simulink model "DDCU_wxt_v02_forA_LabviewV03"  (R2014a)
settings: Solver=FixedStepDiscrete  StartTime=0.0  StopTime=50  FixedStep=0.0005  RelTol=1e-3
InitFcn:
  | Veh_Par_wxt
values from neighbouring files (symbols this model uses):
  ag_thr = 0.4*g    (= 3.924)    [Veh_Par_wxt.m]
  B = 2.25    [Veh_Par_wxt.m]
  bra_pre_em = 12    [Veh_Par_wxt.m]
  bra_pre_gz2 = 12/3    (= 4)    [Veh_Par_wxt.m]
  bra_pre_gz34 = 12/3    (= 4)    [Veh_Par_wxt.m]
  bra_pre_yd = 12/2    (= 6)    [Veh_Par_wxt.m]
  brakepre_dem_data = [0 1 2 3 4 5 6 7 8 9 10 11 12]    [Veh_Par_wxt.m]
  brakeTrq_dem_data = [0 218.198 436.396 654.594 872.792 1090.99 1309.188 1527.386 1745.584 1963.782 2181.98 2400.178 2618.376]    [Veh_Par_wxt.m]
  bratrq_max = 4*2618.376    (= 10473.504)    [Veh_Par_wxt.m]
  eff_tran = 0.75    [Veh_Par_wxt.m]
  G = Mass*g    (= 36297)    [Veh_Par_wxt.m]
  kd1 = 1    [Veh_Par_wxt.m]
  kd2 = 1    [Veh_Par_wxt.m]
  kd3 = 1    [Veh_Par_wxt.m]
  ki1 = 1    [Veh_Par_wxt.m]
  ki2 = 1    [Veh_Par_wxt.m]
  ki3 = 1    [Veh_Par_wxt.m]
  kp1 = 1    [Veh_Par_wxt.m]
  kp2 = 1    [Veh_Par_wxt.m]
  kp3 = 1    [Veh_Par_wxt.m]
  L = 3.12    [Veh_Par_wxt.m]
  premax = 12    [Veh_Par_wxt.m]
  Radius = 0.20    (= 0.2)    [Veh_Par_wxt.m]
  s_opt_yi_add = 0.05    [Veh_Par_wxt.m]
  s_opt_zhuan_add = 0.05    [Veh_Par_wxt.m]
  spd_map_mot = [0 100 200 300 360 400 500 600 700 800 900]*tras_ratio    [Veh_Par_wxt.m]
  spdmax = 900*tras_ratio    (= 5580)    [Veh_Par_wxt.m]
  speed_thr_park = 5/3.6/Radius*30/pi    (= 66.3145596216)    [Veh_Par_wxt.m]
  tras_ratio = 6.2    [Veh_Par_wxt.m]
  trq_map_mot = [1200 1200 1200 1200 1200 1080 864 720 617 540 480]/tras_ratio    [Veh_Par_wxt.m]
  trqmax = 80    [Veh_Par_wxt.m]
  trqmax_yd = 200    [Veh_Par_wxt.m]
  v_thr1_b = 5    [Veh_Par_wxt.m]
  v_thr2_b = 20    [Veh_Par_wxt.m]
  v_thr_park = 5    [Veh_Par_wxt.m]
undefined symbols (not defined in the file or in its folder): DiscIntNeverNeededParam
libraries: simulink x231, ec5744lib x19
(part 4 of 16)

== system DDCU_wxt_v02_forA_LabviewV03/OutputSignalProcess ==
  function : TriggerPort  TriggerType=function-call
  CANTransmit : ec5744lib/RapidECU_U3/04CANCommunication/CANTransmit  canmodule=0  canbuffer=8  canmessageid=hex2dec('0C01F001')  canmessagetype=Extended(29-bit ID)  datalength=8  sampletime=-1
  CANTransmit1 : ec5744lib/RapidECU_U3/04CANCommunication/CANTransmit  canmodule=0  canbuffer=9  canmessageid=hex2dec('0C01F002')  canmessagetype=Extended(29-bit ID)  datalength=8  sampletime=-1
  CANTransmit2 : ec5744lib/RapidECU_U3/04CANCommunication/CANTransmit  Commented=on  canmodule=0  canbuffer=10  canmessageid=hex2dec('804623A')  canmessagetype=Extended(29-bit ID)  datalength=8  sampletime=-1
  CANTransmit3 : ec5744lib/RapidECU_U3/04CANCommunication/CANTransmit  canmodule=0  canbuffer=11  canmessageid=hex2dec('0BF6EAF0')  canmessagetype=Extended(29-bit ID)  datalength=8  sampletime=-1
  Constant{,2..5} (5 alike) : Constant  SampleTime=-1
  Constant1 : Constant  Value=0  SampleTime=-1
  Data Store Read : DataStoreRead  DataStoreName=M1Enable
  Data Store Read1 : DataStoreRead  DataStoreName=M1Mode
  Data Store Read10 : DataStoreRead  DataStoreName=M3Drive
  Data Store Read11 : DataStoreRead  DataStoreName=M3TorqueSet
  Data Store Read12 : DataStoreRead  DataStoreName=M3SpeedSet
  Data Store Read13 : DataStoreRead  DialogController=Simulink.DDGSource  DataStoreName=M3TrqLimit
  Data Store Read14 : DataStoreRead  DataStoreName=M3SpeedLimit
  Data Store Read15 : DataStoreRead  DataStoreName=MCU2HeartBeat
  Data Store Read16 : DataStoreRead  DataStoreName=M2Enable
  Data Store Read17 : DataStoreRead  DataStoreName=M2Mode
  Data Store Read18 : DataStoreRead  DataStoreName=M2Drive
  Data Store Read19 : DataStoreRead  DataStoreName=M2TorqueSet
  Data Store Read2 : DataStoreRead  DataStoreName=M1Drive
  Data Store Read20 : DataStoreRead  DataStoreName=M2SpeedSet
  Data Store Read21 : DataStoreRead  DataStoreName=M2TrqLimit
  Data Store Read22 : DataStoreRead  DataStoreName=M2SpeedLimit
  Data Store Read23 : DataStoreRead  DataStoreName=M4Drive
  Data Store Read24 : DataStoreRead  DataStoreName=M4TorqueSet
  Data Store Read25 : DataStoreRead  DataStoreName=M4SpeedSet
  Data Store Read26 : DataStoreRead  DataStoreName=M4TrqLimit
  Data Store Read27 : DataStoreRead  DataStoreName=M4SpeedLimit
  Data Store Read28 : DataStoreRead  DataStoreName=M4Enable
  Data Store Read29 : DataStoreRead  DataStoreName=M4Mode
  Data Store Read3 : DataStoreRead  DataStoreName=M1TorqueSet
  Data Store Read30 : DataStoreRead  DataStoreName=bra_pre_l
  Data Store Read31 : DataStoreRead  DataStoreName=bra_pre_r
  Data Store Read32 : DataStoreRead  DataStoreName=M1InputVolt
  Data Store Read33 : DataStoreRead  DataStoreName=M4InputVolt
  Data Store Read34 : DataStoreRead  DataStoreName=M2InputVolt
  Data Store Read35 : DataStoreRead  DataStoreName=M3InputVolt
  Data Store Read4 : DataStoreRead  DataStoreName=M1SpeedSet
  Data Store Read5 : DataStoreRead  DataStoreName=M1TrqLimit
  Data Store Read6 : DataStoreRead  DataStoreName=M1SpeedLimit
  Data Store Read7 : DataStoreRead  DataStoreName=MCU1HeartBeat
  Data Store Read8 : DataStoreRead  DataStoreName=M3Enable
  Data Store Read9 : DataStoreRead  DataStoreName=M3Mode
  Data Type Conversion : DataTypeConversion
  Data Type Conversion1 : DataTypeConversion
  Ground : Ground  Commented=on
  Switch{,1..3} (4 alike) : Switch  Criteria=u2 > Threshold  Threshold=330
  Terminator{,1,3..11} (11 alike) : Terminator
  Terminator2 : Terminator  Commented=on
  VCU_ESC : Subsystem
  VCU_MCU1 : Subsystem
  VCU_MCU1_replace : Subsystem  Commented=on
  VCU_MCU2 : Subsystem
  VCU_MCU2_replace : Subsystem  Commented=on
  VCU_Park : Subsystem  Commented=on
  wires:
  Ground/1 -> VCU_Park/1(ParkEnable_in)
  Constant/1 -> Data Type Conversion/1
  VCU_MCU1/1(output) -> CANTransmit/1
  CANTransmit/1 -> Terminator/1
  VCU_MCU2/1(output) -> CANTransmit1/1
  CANTransmit1/1 -> Terminator1/1
  VCU_Park/1(output) -> CANTransmit2/1
  CANTransmit2/1 -> Terminator2/1
  VCU_ESC/1(output) -> CANTransmit3/1
  CANTransmit3/1 -> Terminator3/1
  Data Store Read4/1 -> Terminator4/1
  Data Store Read5/1 -> Terminator5/1
  Data Store Read20/1 -> Terminator6/1
  Data Store Read21/1 -> Terminator7/1
  Data Store Read12/1 -> Terminator8/1
  Data Store Read13/1 -> Terminator9/1
  Data Store Read25/1 -> Terminator10/1
  Data Store Read26/1 -> Terminator11/1
  Data Store Read14/1 -> VCU_MCU2/5(M3SpeedLimit_in)
  Data Store Read11/1 -> VCU_MCU2/4(M3TorqueSet_in)  "M3TorqueSet"
  Data Store Read15/1 -> VCU_MCU2/11(MCU2HeartBeat_in)
  Data Store Read27/1 -> VCU_MCU2/10(M4SpeedLimit_in)
  Data Store Read10/1 -> VCU_MCU2/3(M3Drive_in)  "M3Drive"
  Switch2/1 -> VCU_MCU2/1(M3Enable_in)  "M3Enable1"
  Data Store Read9/1 -> VCU_MCU2/2(M3Mode_in)  "M3Mode"
  Data Store Read24/1 -> VCU_MCU2/9(M4TorqueSet_in)  "M4TorqueSet"
  Data Store Read23/1 -> VCU_MCU2/8(M4Drive_in)  "M4Drive"
  Data Store Read29/1 -> VCU_MCU2/7(M4Mode_in)  "M4Mode"
  Data Store Read31/1 -> VCU_ESC/4(VVMS_BrkPSetRi_MPa_in)  "bra_pre_r"
  Data Store Read30/1 -> VCU_ESC/3(VVMS_BrkPSetLe_MPa_in)  "bra_pre_l"
  Constant1/1 -> Data Type Conversion1/1
  Data Type Conversion/1 -> VCU_ESC/1(VVMS_BrkSts_flg_in)
  Data Type Conversion1/1 -> VCU_ESC/2(VVMS_ParkSts_flg_in)
  Data Store Read7/1 -> VCU_MCU1/11(MCU1HeartBeat_in)
  Data Store Read19/1 -> VCU_MCU1/9(M2TorqueSet_in)  "M2TorqueSet"
  Data Store Read3/1 -> VCU_MCU1/4(M1TorqueSet_in)  "M1TorqueSet"
  Data Store Read6/1 -> VCU_MCU1/5(M1SpeedLimit_in)
  Data Store Read22/1 -> VCU_MCU1/10(M2SpeedLimit_in)
  Switch1/1 -> VCU_MCU1/6(M2Enable_in)  "M2Enable1"
  Data Store Read1/1 -> VCU_MCU1/2(M1Mode_in)  "M1Mode"
  Data Store Read18/1 -> VCU_MCU1/8(M2Drive_in)  "M2Drive"
  Data Store Read2/1 -> VCU_MCU1/3(M1Drive_in)  "M1Drive"
  Data Store Read17/1 -> VCU_MCU1/7(M2Mode_in)  "M2Mode"
  Data Store Read32/1 -> Switch/2
  Constant2/1 -> Switch/3
  Data Store Read/1 -> Switch/1
  Switch/1 -> VCU_MCU1/1(M1Enable_in)  "M1Enable1"
  Data Store Read34/1 -> Switch1/2
  Constant3/1 -> Switch1/3
  Data Store Read16/1 -> Switch1/1
  Data Store Read35/1 -> Switch2/2
  Constant4/1 -> Switch2/3
  Data Store Read8/1 -> Switch2/1
  Data Store Read33/1 -> Switch3/2
  Constant5/1 -> Switch3/3
  Data Store Read28/1 -> Switch3/1
  Switch3/1 -> VCU_MCU2/6(M4Enable_in)  "M4Enable1"

== system DDCU_wxt_v02_forA_LabviewV03/Data_Input/Function-Call Subsystem ==
  In1 : Inport
  In2 : Inport  Port=2
  function : TriggerPort  TriggerType=function-call
  ddcu1_ddcu2 : Subsystem
  brake_emerg : Outport
  steer_dem : Outport  Port=2
  mode_dem : Outport  Port=3
  brake_dem : Outport  Port=4
  acc_dem : Outport  Port=5
  wires:
  In1/1 -> ddcu1_ddcu2/Enable
  In2/1 -> ddcu1_ddcu2/1(input)
  ddcu1_ddcu2/3(mode_dem_Out) -> mode_dem/1
  ddcu1_ddcu2/2(steer_dem_Out) -> steer_dem/1
  ddcu1_ddcu2/4(brake_dem_Out) -> brake_dem/1
  ddcu1_ddcu2/1(brake_emerg_Out) -> brake_emerg/1
  ddcu1_ddcu2/5(acc_dem_Out) -> acc_dem/1

== system DDCU_wxt_v02_forA_LabviewV03/Data_Input/Function-Call Subsystem2 ==
  In1 : Inport
  In2 : Inport  Port=2
  function : TriggerPort  TriggerType=function-call
  ESC_VCU : Subsystem
  VESC_BrkPMa_MPa : Outport
  VESC_BrkPSetRi_MPa : Outport  Port=2
  VESC_BrkPSetLe_MPa : Outport  Port=3
  VESC_BrkFlt_enum : Outport  Port=4
  VESC_HotSts_flg : Outport  Port=5
  VESC_BrkReq_flg : Outport  Port=6
  VESC_ParkReq_flg : Outport  Port=7
  VESC_BrkPRi_MPa : Outport  Port=8
  VESC_BrkPLe_MPa : Outport  Port=9
  wires:
  ESC_VCU/1(VESC_BrkPMa_MPa_Out) -> VESC_BrkPMa_MPa/1
  ESC_VCU/2(VESC_BrkPSetRi_MPa_Out) -> VESC_BrkPSetRi_MPa/1
  ESC_VCU/3(VESC_BrkPSetLe_MPa_Out) -> VESC_BrkPSetLe_MPa/1
  ESC_VCU/4(VESC_BrkFlt_enum_Out) -> VESC_BrkFlt_enum/1
  ESC_VCU/5(VESC_HotSts_flg_Out) -> VESC_HotSts_flg/1
  ESC_VCU/6(VESC_BrkReq_flg_Out) -> VESC_BrkReq_flg/1
  ESC_VCU/7(VESC_ParkReq_flg_Out) -> VESC_ParkReq_flg/1
  ESC_VCU/8(VESC_BrkPRi_MPa_Out) -> VESC_BrkPRi_MPa/1
  ESC_VCU/9(VESC_BrkPLe_MPa_Out) -> VESC_BrkPLe_MPa/1
  In2/1 -> ESC_VCU/1(input)
  In1/1 -> ESC_VCU/Enable

== system DDCU_wxt_v02_forA_LabviewV03/Data_Input/HCU1_VCU ==
  In1 : Inport
  In2 : Inport  Port=2
  function : TriggerPort  TriggerType=function-call
  HCU1_VCU : Subsystem
  turn : Outport
  real_velocity : Outport  Port=2
  pwr_limit : Outport  Port=3
  break : Outport  Port=4
  acc : Outport  Port=5
  wires:
  In1/1 -> HCU1_VCU/Enable
  In2/1 -> HCU1_VCU/1(input)
  HCU1_VCU/3(pwr_limit_Out) -> pwr_limit/1
  HCU1_VCU/4(break_Out) -> break/1
  HCU1_VCU/2(real_velocity_Out) -> real_velocity/1
  HCU1_VCU/5(acc_Out) -> acc/1
  HCU1_VCU/1(turn_Out) -> turn/1

== system DDCU_wxt_v02_forA_LabviewV03/Data_Input/HCU1_VCU1 ==
  In1 : Inport
  In2 : Inport  Port=2
  function : TriggerPort  TriggerType=function-call
  MUC1_VCU1 : Subsystem
  spd_mot_rr : Outport
  spd_mot_rf : Outport  Port=2
  spd_mot_lr : Outport  Port=3
  spd_mot_lf : Outport  Port=4
  wires:
  In2/1 -> MUC1_VCU1/1(input)
  In1/1 -> MUC1_VCU1/Enable
  MUC1_VCU1/2(spd_mot_rf_Out) -> spd_mot_rf/1
  MUC1_VCU1/1(spd_mot_rr_Out) -> spd_mot_rr/1
  MUC1_VCU1/3(spd_mot_lr_Out) -> spd_mot_lr/1
  MUC1_VCU1/4(spd_mot_lf_Out) -> spd_mot_lf/1

== system DDCU_wxt_v02_forA_LabviewV03/Data_Input/HCU2_VCU ==
  In1 : Inport
  In2 : Inport  Port=2
  function : TriggerPort  TriggerType=function-call
  HCU2_VCU : Subsystem
  zhuche : Outport
  zhongxinzhuanxiang : Outport  Port=2
  qianjin : Outport  Port=3
  kongdang : Outport  Port=4
  daodang : Outport  Port=5
  wires:
  In2/1 -> HCU2_VCU/1(input)
  In1/1 -> HCU2_VCU/Enable
  HCU2_VCU/2(zhongxinzhuanxiang_Out) -> zhongxinzhuanxiang/1
  HCU2_VCU/3(qianjin_Out) -> qianjin/1
  HCU2_VCU/1(zhuche_Out) -> zhuche/1
  HCU2_VCU/4(kongdang_Out) -> kongdang/1
  HCU2_VCU/5(daodang_Out) -> daodang/1

== system DDCU_wxt_v02_forA_LabviewV03/Data_Input/MCU1_VCU1 ==
  In1 : Inport
  In2 : Inport  Port=2
  function : TriggerPort  TriggerType=function-call
  MCU1_VCU1 : Subsystem
  M1InputVolt : Outport
  M1Speed : Outport  Port=2
  M1Direction : Outport  Port=3
  M1State : Outport  Port=4
  M1HeartBeat : Outport  Port=5
  M1Current : Outport  Port=6
  M1Torque : Outport  Port=7
  wires:
  In1/1 -> MCU1_VCU1/Enable
  MCU1_VCU1/2(M1Speed_Out) -> M1Speed/1
  MCU1_VCU1/3(M1Direction_Out) -> M1Direction/1
  MCU1_VCU1/4(M1State_Out) -> M1State/1
  MCU1_VCU1/1(M1InputVolt_Out) -> M1InputVolt/1
  MCU1_VCU1/5(M1HeartBeat_Out) -> M1HeartBeat/1
  MCU1_VCU1/6(M1Current_Out) -> M1Current/1
  MCU1_VCU1/7(M1Torque_Out) -> M1Torque/1
  In2/1 -> MCU1_VCU1/1(input)

== system DDCU_wxt_v02_forA_LabviewV03/Data_Input/MCU1_VCU2 ==
  In1 : Inport
  In2 : Inport  Port=2
  function : TriggerPort  TriggerType=function-call
  MCU1_VCU2 : Subsystem
  M1FaultGrade : Outport
  M1FaultCode : Outport  Port=2
  M1TqLimit : Outport  Port=3
  M1IGBTTemp : Outport  Port=4
  M1Temp : Outport  Port=5
  wires:
  In1/1 -> MCU1_VCU2/Enable
  In2/1 -> MCU1_VCU2/1(input)
  MCU1_VCU2/2(M1FaultCode_Out) -> M1FaultCode/1
  MCU1_VCU2/3(M1TqLimit_Out) -> M1TqLimit/1
  MCU1_VCU2/1(M1FaultGrade_Out) -> M1FaultGrade/1
  MCU1_VCU2/4(M1IGBTTemp_Out) -> M1IGBTTemp/1
  MCU1_VCU2/5(M1Temp_Out) -> M1Temp/1

== system DDCU_wxt_v02_forA_LabviewV03/Data_Input/MCU1_VCU3 ==
  In1 : Inport
  In2 : Inport  Port=2
  function : TriggerPort  TriggerType=function-call
  MCU1_VCU3 : Subsystem
  M2InputVolt : Outport
  M2Speed : Outport  Port=2
  M2Direction : Outport  Port=3
  M2State : Outport  Port=4
  M2HeartBeat : Outport  Port=5
  M2Current : Outport  Port=6
  M2Torque : Outport  Port=7
  wires:
  In2/1 -> MCU1_VCU3/1(input)
  In1/1 -> MCU1_VCU3/Enable
  MCU1_VCU3/3(M2Direction_Out) -> M2Direction/1
  MCU1_VCU3/6(M2Current_Out) -> M2Current/1
  MCU1_VCU3/5(M2HeartBeat_Out) -> M2HeartBeat/1
  MCU1_VCU3/1(M2InputVolt_Out) -> M2InputVolt/1
  MCU1_VCU3/2(M2Speed_Out) -> M2Speed/1
  MCU1_VCU3/4(M2State_Out) -> M2State/1
  MCU1_VCU3/7(M2Torque_Out) -> M2Torque/1

== system DDCU_wxt_v02_forA_LabviewV03/Data_Input/MCU1_VCU4 ==
  In1 : Inport
  In2 : Inport  Port=2
  function : TriggerPort  TriggerType=function-call
  MCU1_VCU4 : Subsystem
  M2FaultGrade : Outport
  M2FaultCode : Outport  Port=2
  M2TqLimit : Outport  Port=3
  M2IGBTTemp : Outport  Port=4
  M2Temp : Outport  Port=5
  wires:
  In1/1 -> MCU1_VCU4/Enable
  In2/1 -> MCU1_VCU4/1(input)
  MCU1_VCU4/5(M2Temp_Out) -> M2Temp/1
  MCU1_VCU4/4(M2IGBTTemp_Out) -> M2IGBTTemp/1
  MCU1_VCU4/3(M2TqLimit_Out) -> M2TqLimit/1
  MCU1_VCU4/1(M2FaultGrade_Out) -> M2FaultGrade/1
  MCU1_VCU4/2(M2FaultCode_Out) -> M2FaultCode/1

== system DDCU_wxt_v02_forA_LabviewV03/Data_Input/MCU2_VCU1 ==
  In1 : Inport
  In2 : Inport  Port=2
  function : TriggerPort  TriggerType=function-call
  MCU2_VCU1 : Subsystem
  M3InputVolt : Outport
  M3Speed : Outport  Port=2
  M3Direction : Outport  Port=3
  M3State : Outport  Port=4
  M3HeartBeat : Outport  Port=5
  M3Current : Outport  Port=6
  M3Torque : Outport  Port=7
  wires:
  In1/1 -> MCU2_VCU1/Enable
  In2/1 -> MCU2_VCU1/1(input)
  MCU2_VCU1/7(M3Torque_Out) -> M3Torque/1
  MCU2_VCU1/6(M3Current_Out) -> M3Current/1
  MCU2_VCU1/5(M3HeartBeat_Out) -> M3HeartBeat/1
  MCU2_VCU1/4(M3State_Out) -> M3State/1
  MCU2_VCU1/3(M3Direction_Out) -> M3Direction/1
  MCU2_VCU1/2(M3Speed_Out) -> M3Speed/1
  MCU2_VCU1/1(M3InputVolt_Out) -> M3InputVolt/1

== system DDCU_wxt_v02_forA_LabviewV03/Data_Input/MCU2_VCU2 ==
  In1 : Inport
  In2 : Inport  Port=2
  function : TriggerPort  TriggerType=function-call
  MCU2_VCU2 : Subsystem
  M3FaultGrade : Outport
  M3FaultCode : Outport  Port=2
  M3TqLimit : Outport  Port=3
  M3IGBTTemp : Outport  Port=4
  M3Temp : Outport  Port=5
  wires:
  In1/1 -> MCU2_VCU2/Enable
  In2/1 -> MCU2_VCU2/1(input)
  MCU2_VCU2/2(M3FaultCode_Out) -> M3FaultCode/1
  MCU2_VCU2/1(M3FaultGrade_Out) -> M3FaultGrade/1
  MCU2_VCU2/3(M3TqLimit_Out) -> M3TqLimit/1
  MCU2_VCU2/4(M3IGBTTemp_Out) -> M3IGBTTemp/1
  MCU2_VCU2/5(M3Temp_Out) -> M3Temp/1

== system DDCU_wxt_v02_forA_LabviewV03/Data_Input/MCU2_VCU3 ==
  In1 : Inport
  In2 : Inport  Port=2
  function : TriggerPort  TriggerType=function-call
  MCU2_VCU3 : Subsystem
  M4InputVolt : Outport
  M4Speed : Outport  Port=2
  M4Direction : Outport  Port=3
  M4State : Outport  Port=4
  M4HeartBeat : Outport  Port=5
  M4Current : Outport  Port=6
  M4Torque : Outport  Port=7
  wires:
  In1/1 -> MCU2_VCU3/Enable
  In2/1 -> MCU2_VCU3/1(input)
  MCU2_VCU3/2(M4Speed_Out) -> M4Speed/1
  MCU2_VCU3/3(M4Direction_Out) -> M4Direction/1
  MCU2_VCU3/1(M4InputVolt_Out) -> M4InputVolt/1
  MCU2_VCU3/4(M4State_Out) -> M4State/1
  MCU2_VCU3/5(M4HeartBeat_Out) -> M4HeartBeat/1
  MCU2_VCU3/6(M4Current_Out) -> M4Current/1
  MCU2_VCU3/7(M4Torque_Out) -> M4Torque/1

== system DDCU_wxt_v02_forA_LabviewV03/Data_Input/MCU2_VCU4 ==
  In1 : Inport
  In2 : Inport  Port=2
  function : TriggerPort  TriggerType=function-call
  MCU2_VCU4 : Subsystem
  M4FaultGrade : Outport
  M4FaultCode : Outport  Port=2
  M4TqLimit : Outport  Port=3
  M4IGBTTemp : Outport  Port=4
  M4Temp : Outport  Port=5
  wires:
  In1/1 -> MCU2_VCU4/Enable
  In2/1 -> MCU2_VCU4/1(input)
  MCU2_VCU4/5(M4Temp_Out) -> M4Temp/1
  MCU2_VCU4/4(M4IGBTTemp_Out) -> M4IGBTTemp/1
  MCU2_VCU4/3(M4TqLimit_Out) -> M4TqLimit/1
  MCU2_VCU4/1(M4FaultGrade_Out) -> M4FaultGrade/1
  MCU2_VCU4/2(M4FaultCode_Out) -> M4FaultCode/1

== system DDCU_wxt_v02_forA_LabviewV03/InputSignalProcess/Battery ==
  pwr_dis_bat : Inport
  pwr_chg_bat : Inport  Port=2
  Bus Creator : BusCreator  Inputs=2
  Bat : Outport
  wires:
  pwr_dis_bat/1 -> Bus Creator/1  "pwr_dis_bat"
  Bus Creator/1 -> Bat/1  "Bat"
  pwr_chg_bat/1 -> Bus Creator/2  "pwr_chg_bat"

== system DDCU_wxt_v02_forA_LabviewV03/InputSignalProcess/BraSystem ==
  BraPre_act_l : Inport
  BraPre_act_r : Inport  Port=2
  Bus Creator : BusCreator  Inputs=2
  BraPre : Outport
  wires:
  BraPre_act_l/1 -> Bus Creator/1  "BraPre_act"
  Bus Creator/1 -> BraPre/1  "BraPre"
  BraPre_act_r/1 -> Bus Creator/2  "BraPre_act_r"

== system DDCU_wxt_v02_forA_LabviewV03/InputSignalProcess/DriveMotor ==
  speed_act_lf : Inport
  trq_act_lf : Inport  Port=2
  trqlimU_dig_lf : Inport  Port=3
  trqlimL_dig_lf : Inport  Port=4
  guzhang_lf : Inport  Port=5
  speed_act_lr : Inport  Port=6
  trq_act_lr : Inport  Port=7
  trqlimU_dig_lr : Inport  Port=8
  trqlimL_dig_lr : Inport  Port=9
  guzhang_lr : Inport  Port=10
  speed_act_rf : Inport  Port=11
  trq_act_rf : Inport  Port=12
  trqlimU_dig_rf : Inport  Port=13
  trqlimL_dig_rf : Inport  Port=14
  guzhang_rf : Inport  Port=15
  speed_act_rr : Inport  Port=16
  trq_act_rr : Inport  Port=17
  trqlimU_dig_rr : Inport  Port=18
  trqlimL_dig_rr : Inport  Port=19
  guzhang_rr : Inport  Port=20
  Bus Creator : BusCreator  Inputs=20
  DriveMotor : Outport
  wires:
  Bus Creator/1 -> DriveMotor/1  "DriveMotor"
  trqlimL_dig_lr/1 -> Bus Creator/9  "trqlimL_dig_lr"
  trq_act_lf/1 -> Bus Creator/2  "trq_act_lf"
  trq_act_lr/1 -> Bus Creator/7  "trq_act_lr"
  trqlimL_dig_lf/1 -> Bus Creator/4  "trqlimL_dig_lf"
  trqlimU_dig_lf/1 -> Bus Creator/3  "trqlimU_dig_lf"
  trqlimU_dig_lr/1 -> Bus Creator/8  "trqlimU_dig_lr"
  speed_act_lf/1 -> Bus Creator/1  "speed_act_lf"
  speed_act_lr/1 -> Bus Creator/6  "speed_act_lr"
  guzhang_rf/1 -> Bus Creator/15  "guzhang_rf"
  guzhang_lf/1 -> Bus Creator/5  "guzhang_lf"
  guzhang_lr/1 -> Bus Creator/10  "guzhang_lr"
  speed_act_rf/1 -> Bus Creator/11  "speed_act_rf"
  guzhang_rr/1 -> Bus Creator/20  "guzhang_rr"
  trq_act_rf/1 -> Bus Creator/12  "trq_act_rf"
  speed_act_rr/1 -> Bus Creator/16  "speed_act_rr"
  trqlimL_dig_rf/1 -> Bus Creator/14  "trqlimL_dig_rf"
  trq_act_rr/1 -> Bus Creator/17  "trq_act_rr"
  trqlimL_dig_rr/1 -> Bus Creator/19  "trqlimL_dig_rr"
  trqlimU_dig_rf/1 -> Bus Creator/13  "trqlimU_dig_rf"
  trqlimU_dig_rr/1 -> Bus Creator/18  "trqlimU_dig_rr"

== system DDCU_wxt_v02_forA_LabviewV03/InputSignalProcess/IMU ==
  v_act : Inport
  dis_east : Inport  Port=2
  dis_north : Inport  Port=3
  dis_sky : Inport  Port=4
  hangxiangangle : Inport  Port=5
  fuyangangle : Inport  Port=6
  henggunangle : Inport  Port=7
  acc_x : Inport  Port=8
  acc_y : Inport  Port=9
  acc_z : Inport  Port=10
  jiaosudu_x : Inport  Port=11
  jiaosudu_y : Inport  Port=12
  jiaosudu_z : Inport  Port=13
  Bus Creator : BusCreator  Inputs=13
  IMU : Outport
  wires:
  Bus Creator/1 -> IMU/1  "IMU"
  dis_east/1 -> Bus Creator/2  "dis_east"
  hangxiangangle/1 -> Bus Creator/5  "hangxiangangle"
  dis_north/1 -> Bus Creator/3  "dis_north"
  dis_sky/1 -> Bus Creator/4  "dis_sky"
  fuyangangle/1 -> Bus Creator/6  "fuyangangle"
  acc_y/1 -> Bus Creator/9  "acc_y"
  henggunangle/1 -> Bus Creator/7  "henggunangle"
  acc_x/1 -> Bus Creator/8  "acc_x"
  acc_z/1 -> Bus Creator/10  "acc_z"
  jiaosudu_z/1 -> Bus Creator/13  "jiaosudu_z"
  jiaosudu_x/1 -> Bus Creator/11  "jiaosudu_x"
  jiaosudu_y/1 -> Bus Creator/12  "jiaosudu_y"
  v_act/1 -> Bus Creator/1  "v_act"

== system DDCU_wxt_v02_forA_LabviewV03/InputSignalProcess/Subsystem ==
  zhuche : Inport
  zhongxinzhuanxiang : Inport  Port=2
  qianjin : Inport  Port=3
  kongdang : Inport  Port=4
  daodang : Inport  Port=5
  MATLAB Function : MATLAB Function  TreatAsAtomicUnit=on
  mode_dem : Outport
  wires:
  MATLAB Function/1(mode_dem) -> mode_dem/1
  zhuche/1 -> MATLAB Function/1(zhuche)
  zhongxinzhuanxiang/1 -> MATLAB Function/2(zhongxinzhuanxiang)
  qianjin/1 -> MATLAB Function/3(qianjin)
  kongdang/1 -> MATLAB Function/4(kongdang)
  daodang/1 -> MATLAB Function/5(daodang)

== system DDCU_wxt_v02_forA_LabviewV03/InputSignalProcess/Suspension ==
  location_center : Inport
  Bus Creator : BusCreator  Inputs=1
  Center_of_Mass : Outport
  wires:
  Bus Creator/1 -> Center_of_Mass/1  "Center_of_Mass"
  location_center/1 -> Bus Creator/1  "location_center"

== system DDCU_wxt_v02_forA_LabviewV03/InputSignalProcess/YaoKong ==
  note: 上坡辅助系统(Hill-start Assist Control，HAC)
  mode_dem : Inport
  acc_dem : Inport  Port=2
  steer_dem : Inport  Port=3
  brake_dem : Inport  Port=4
  brake_emerg : Inport  Port=5
  HAC : Inport  Port=6
  Bus Creator : BusCreator  Inputs=6
  YaoKong_dem : Outport
  wires:
  steer_dem/1 -> Bus Creator/3  "steer_dem"
  acc_dem/1 -> Bus Creator/2  "acc_dem"
  brake_dem/1 -> Bus Creator/4  "brake_dem"
  mode_dem/1 -> Bus Creator/1  "mode_dem"
  Bus Creator/1 -> YaoKong_dem/1  "YaoKong"
  brake_emerg/1 -> Bus Creator/5  "brake_emerg"
  HAC/1 -> Bus Creator/6  "HAC"

== system DDCU_wxt_v02_forA_LabviewV03/MainControl/SendOutPrepare ==
  com_dem : Inport
  Data Store Write : DataStoreWrite  DataStoreName=M1Enable
  Data Store Write1 : DataStoreWrite  DataStoreName=M1Mode
  Data Store Write10 : DataStoreWrite  DataStoreName=M3Drive
  Data Store Write11 : DataStoreWrite  DataStoreName=M3TorqueSet
  Data Store Write12 : DataStoreWrite  DataStoreName=M3SpeedSet
  Data Store Write13 : DataStoreWrite  DialogController=Simulink.DDGSource  DataStoreName=M3TrqLimit
  Data Store Write14 : DataStoreWrite  DataStoreName=M3SpeedLimit
  Data Store Write15 : DataStoreWrite  DataStoreName=MCU2HeartBeat
  Data Store Write16 : DataStoreWrite  DataStoreName=M2Enable
  Data Store Write17 : DataStoreWrite  DataStoreName=M2Mode
  Data Store Write18 : DataStoreWrite  DataStoreName=M2Drive
  Data Store Write19 : DataStoreWrite  DataStoreName=M2TorqueSet
  Data Store Write2 : DataStoreWrite  DataStoreName=M1Drive
  Data Store Write20 : DataStoreWrite  DataStoreName=M2SpeedSet
  Data Store Write21 : DataStoreWrite  DataStoreName=M2TrqLimit
  Data Store Write22 : DataStoreWrite  DataStoreName=M2SpeedLimit
  Data Store Write23 : DataStoreWrite  DataStoreName=M4Drive
  Data Store Write24 : DataStoreWrite  DataStoreName=M4TorqueSet
  Data Store Write25 : DataStoreWrite  DataStoreName=M4SpeedSet
  Data Store Write26 : DataStoreWrite  DataStoreName=M4TrqLimit
  Data Store Write27 : DataStoreWrite  DataStoreName=M4SpeedLimit
  Data Store Write28 : DataStoreWrite  DataStoreName=M4Enable
  Data Store Write29 : DataStoreWrite  DataStoreName=M4Mode
  Data Store Write3 : DataStoreWrite  DataStoreName=M1TorqueSet
  Data Store Write30 : DataStoreWrite  DataStoreName=bra_pre_l
  Data Store Write31 : DataStoreWrite  DataStoreName=bra_pre_r
  Data Store Write4 : DataStoreWrite  DataStoreName=M1SpeedSet
  Data Store Write5 : DataStoreWrite  DataStoreName=M1TrqLimit
  Data Store Write6 : DataStoreWrite  DataStoreName=M1SpeedLimit
  Data Store Write7 : DataStoreWrite  DataStoreName=MCU1HeartBeat
  Data Store Write8 : DataStoreWrite  DataStoreName=M3Enable
  Data Store Write9 : DataStoreWrite  DataStoreName=M3Mode
  Demux : Demux  Outputs=6
  Demux1 : Demux  Outputs=8
  Demux2 : Demux  Outputs=8
  Demux3 : Demux  Outputs=7
  Demux4 : Demux  Outputs=7
  Scope{,1..3} (4 alike) : Scope
      Scope2 settings: SaveName=ScopeData2
      Scope3 settings: SaveName=ScopeData3
  wires:
  Demux/1 -> Demux1/1
  Demux/2 -> Demux2/1
  Demux/3 -> Demux3/1
  Demux/4 -> Demux4/1
  Demux1/3 -> Data Store Write2/1
  Demux1/4 -> Scope/1, Data Store Write3/1
  Demux1/2 -> Data Store Write1/1
  Demux1/5 -> Data Store Write4/1
  Demux1/6 -> Data Store Write5/1
  Demux1/1 -> Data Store Write/1
  Demux1/7 -> Data Store Write6/1
  Demux1/8 -> Data Store Write7/1
  Demux2/7 -> Data Store Write14/1
  Demux2/6 -> Data Store Write13/1
  Demux2/1 -> Data Store Write8/1
  Demux2/8 -> Data Store Write15/1
  Demux2/5 -> Data Store Write12/1
  Demux2/2 -> Data Store Write9/1
  Demux2/4 -> Scope1/1, Data Store Write11/1
  Demux2/3 -> Data Store Write10/1
  Demux3/1 -> Data Store Write16/1
  Demux3/6 -> Data Store Write21/1
  Demux3/7 -> Data Store Write22/1
  Demux3/5 -> Data Store Write20/1
  Demux3/4 -> Scope2/1, Data Store Write19/1
  Demux3/2 -> Data Store Write17/1
  Demux3/3 -> Data Store Write18/1
  Demux4/1 -> Data Store Write28/1
  Demux4/2 -> Data Store Write29/1
  Demux4/3 -> Data Store Write23/1
  Demux4/4 -> Scope3/1, Data Store Write24/1
  Demux4/5 -> Data Store Write25/1
  Demux4/6 -> Data Store Write26/1
  Demux4/7 -> Data Store Write27/1
  Demux/5 -> Data Store Write30/1
  Demux/6 -> Data Store Write31/1
  com_dem/1 -> Demux/1

== system DDCU_wxt_v02_forA_LabviewV03/MainControl/mode_control ==
  mode_dem_out : Inport
  Signals : Inport  Port=2
  Multiport Switch : MultiPortSwitch  DataPortOrder=Zero-based contiguous  Inputs=6
  Park : Subsystem  TreatAsAtomicUnit=on
  Switch Case : SwitchCase  CaseConditions={0,1,2,3,4,5}  ShowDefaultCase=off
  backward : Subsystem  TreatAsAtomicUnit=on
  center_steer : Subsystem  TreatAsAtomicUnit=on
  emergency_stop : Subsystem  TreatAsAtomicUnit=on
  forward : Subsystem  TreatAsAtomicUnit=on
  neutral : Subsystem  TreatAsAtomicUnit=on
  com_dem : Outport
  wires:
  mode_dem_out/1 -> Multiport Switch/1, Switch Case/1  "mode_dem_out"
  Signals/1 -> backward/1(Signals), emergency_stop/1(Signals), center_steer/1(Signals), neutral/1(Signals), forward/1(Signals), Park/1(Signals)
  Switch Case/1 -> Park/Action
  Switch Case/6 -> emergency_stop/Action
  Switch Case/5 -> center_steer/Action
  Switch Case/4 -> backward/Action
  Switch Case/3 -> neutral/Action
  Switch Case/2 -> forward/Action
  Park/1(park_dem) -> Multiport Switch/2
  forward/1(forward_dem) -> Multiport Switch/3
  backward/1(backward_dem) -> Multiport Switch/5
  neutral/1(neutral_dem) -> Multiport Switch/4
  center_steer/1(center_steer_dem) -> Multiport Switch/6
  emergency_stop/1(emergency_stop_dem) -> Multiport Switch/7
  Multiport Switch/1 -> com_dem/1

== system DDCU_wxt_v02_forA_LabviewV03/MainControl/mode_switch ==
  note: 驻车转速
  note: 驻车车速阈值5km/h
  Signals : Inport
  Abs{,1..3} (4 alike) : Abs
  Bus Selector : BusSelector  OutputSignals=YaoKong.mode_dem,YaoKong.brake_emerg,DriveMotor.speed_act_lf,DriveMotor.speed_act_lr,DriveMotor.speed_act_rf,DriveMotor.speed_act_rr,IMU.v_act
  Constant1 : Constant  Value=v_thr_park  SampleTime=-1
  Constant2 : Constant  Value=speed_thr_park  SampleTime=-1
  Data Type Conversion : DataTypeConversion
  Data Type Conversion1 : DataTypeConversion
  Data Type Conversion2 : DataTypeConversion
  Memory : Memory  InheritSampleTime=on
  mode_switch : MATLAB Function  TreatAsAtomicUnit=on
  mode_dem_out : Outport
  wires:
  Memory/1 -> mode_switch/10(mode_dem_out_pre)
  Signals/1 -> Data Type Conversion/1
  Bus Selector/3 -> Abs/1  "<speed_act_lf>"
  Bus Selector/2 -> mode_switch/2(brake_emerg)  "<brake_emerg>"
  Bus Selector/1 -> mode_switch/1(mode_dem)  "<mode_dem>"
  Bus Selector/5 -> Abs2/1  "<speed_act_rf>"
  Bus Selector/4 -> Abs1/1  "<speed_act_lr>"
  Bus Selector/6 -> Abs3/1  "<speed_act_rr>"
  Bus Selector/7 -> mode_switch/7(v_act)  "<v_act>"
  mode_switch/1(mode_dem_out) -> mode_dem_out/1, Memory/1
  Constant2/1 -> Data Type Conversion2/1
  Constant1/1 -> Data Type Conversion1/1
  Abs/1 -> mode_switch/3(speed_act_lf)
  Abs1/1 -> mode_switch/4(speed_act_lr)
  Abs2/1 -> mode_switch/5(speed_act_rf)
  Abs3/1 -> mode_switch/6(speed_act_rr)
  Data Type Conversion/1 -> Bus Selector/1
  Data Type Conversion1/1 -> mode_switch/8(v_thr_park)
  Data Type Conversion2/1 -> mode_switch/9(speed_thr_park)

== system DDCU_wxt_v02_forA_LabviewV03/OutputSignalProcess/VCU_ESC ==
  VVMS_BrkSts_flg_in : Inport
  VVMS_ParkSts_flg_in : Inport  Port=2
  VVMS_BrkPSetLe_MPa_in : Inport  Port=3
  VVMS_BrkPSetRi_MPa_in : Inport  Port=4
  Conv{1..8} (8 alike) : DataTypeConversion
  VCU_ESC_DLC : Constant  Value=8  OutDataTypeStr=uint8
  VCU_ESC_DLC_Out : Terminator
  VCU_ESC_ID : Constant  Value=2364992240  OutDataTypeStr=single
  VCU_ESC_ID_Out : Terminator
  VCU_ESC_mux : Mux  Inputs=8
  VVMS_BrkPSetLe_MPa : Subsystem
  VVMS_BrkPSetRi_MPa : Subsystem
  VVMS_BrkSts_flg : Subsystem
  VVMS_ParkSts_flg : Subsystem
  or{1..8} (8 alike) : simulink/Logic and Bit Operations/Bitwise Operator  logicop=OR  UseBitMask=off  NumInputPorts=4  BitMask=bin2dec('11011001')  BitMaskRealWorld=Stored Integer
  output : Outport
  wires:
  VCU_ESC_mux/1 -> output/1
  VVMS_BrkSts_flg/1(output1) -> or1/1
  VVMS_BrkSts_flg/2(output2) -> or2/1
  VVMS_BrkSts_flg/3(output3) -> or3/1
  VVMS_BrkSts_flg/4(output4) -> or4/1
  VVMS_BrkSts_flg/5(output5) -> or5/1
  VVMS_BrkSts_flg/6(output6) -> or6/1
  VVMS_BrkSts_flg/7(output7) -> or7/1
  VVMS_BrkSts_flg/8(output8) -> or8/1
  VVMS_ParkSts_flg/1(output1) -> or1/2
  VVMS_ParkSts_flg/2(output2) -> or2/2
  VVMS_ParkSts_flg/3(output3) -> or3/2
  VVMS_ParkSts_flg/4(output4) -> or4/2
  VVMS_ParkSts_flg/5(output5) -> or5/2
  VVMS_ParkSts_flg/6(output6) -> or6/2
  VVMS_ParkSts_flg/7(output7) -> or7/2
  VVMS_ParkSts_flg/8(output8) -> or8/2
  VVMS_BrkPSetRi_MPa/1(output1) -> or1/3
  VVMS_BrkPSetRi_MPa/2(output2) -> or2/3
  VVMS_BrkPSetRi_MPa/3(output3) -> or3/3
  VVMS_BrkPSetRi_MPa/4(output4) -> or4/3
  VVMS_BrkPSetRi_MPa/5(output5) -> or5/3
  VVMS_BrkPSetRi_MPa/6(output6) -> or6/3
  VVMS_BrkPSetRi_MPa/7(output7) -> or7/3
  VVMS_BrkPSetRi_MPa/8(output8) -> or8/3
  VVMS_BrkPSetLe_MPa/1(output1) -> or1/4
  VVMS_BrkPSetLe_MPa/2(output2) -> or2/4
  VVMS_BrkPSetLe_MPa/3(output3) -> or3/4
  VVMS_BrkPSetLe_MPa/4(output4) -> or4/4
  VVMS_BrkPSetLe_MPa/5(output5) -> or5/4
  VVMS_BrkPSetLe_MPa/6(output6) -> or6/4
  VVMS_BrkPSetLe_MPa/7(output7) -> or7/4
  VVMS_BrkPSetLe_MPa/8(output8) -> or8/4
  or1/1 -> Conv1/1
  Conv1/1 -> VCU_ESC_mux/1
  or2/1 -> Conv2/1
  Conv2/1 -> VCU_ESC_mux/2
  or3/1 -> Conv3/1
  Conv3/1 -> VCU_ESC_mux/3
  or4/1 -> Conv4/1
  Conv4/1 -> VCU_ESC_mux/4
  or5/1 -> Conv5/1
  Conv5/1 -> VCU_ESC_mux/5
  or6/1 -> Conv6/1
  Conv6/1 -> VCU_ESC_mux/6
  or7/1 -> Conv7/1
  Conv7/1 -> VCU_ESC_mux/7
  or8/1 -> Conv8/1
  Conv8/1 -> VCU_ESC_mux/8
  VCU_ESC_ID/1 -> VCU_ESC_ID_Out/1
  VCU_ESC_DLC/1 -> VCU_ESC_DLC_Out/1
  VVMS_BrkSts_flg_in/1 -> VVMS_BrkSts_flg/1(VVMS_BrkSts_flg)
  VVMS_ParkSts_flg_in/1 -> VVMS_ParkSts_flg/1(VVMS_ParkSts_flg)
  VVMS_BrkPSetRi_MPa_in/1 -> VVMS_BrkPSetRi_MPa/1(VVMS_BrkPSetRi_MPa)
  VVMS_BrkPSetLe_MPa_in/1 -> VVMS_BrkPSetLe_MPa/1(VVMS_BrkPSetLe_MPa)

== system DDCU_wxt_v02_forA_LabviewV03/OutputSignalProcess/VCU_MCU1 ==
  M1Enable_in : Inport
  M1Mode_in : Inport  Port=2
  M1Drive_in : Inport  Port=3
  M1TorqueSet_in : Inport  Port=4
  M1SpeedLimit_in : Inport  Port=5
  M2Enable_in : Inport  Port=6
  M2Mode_in : Inport  Port=7
  M2Drive_in : Inport  Port=8
  M2TorqueSet_in : Inport  Port=9
  M2SpeedLimit_in : Inport  Port=10
  MCU1HeartBeat_in : Inport  Port=11
  Conv{1..8} (8 alike) : DataTypeConversion
  M1Drive : Subsystem
  M1Enable : Subsystem
  M1Mode : Subsystem
  M1SpeedLimit : Subsystem
  M1TorqueSet : Subsystem
  M2Drive : Subsystem
  M2Enable : Subsystem
  M2Mode : Subsystem
  M2SpeedLimit : Subsystem
  M2TorqueSet : Subsystem
  MCU1HeartBeat : Subsystem
  VCU_MCU1_DLC : Constant  Value=8  OutDataTypeStr=uint8
  VCU_MCU1_DLC_Out : Terminator
  VCU_MCU1_ID : Constant  Value=2348937217  OutDataTypeStr=single
  VCU_MCU1_ID_Out : Terminator
  VCU_MCU1_mux : Mux  Inputs=8
  or{1..8} (8 alike) : simulink/Logic and Bit Operations/Bitwise Operator  logicop=OR  UseBitMask=off  NumInputPorts=11  BitMask=bin2dec('11011001')  BitMaskRealWorld=Stored Integer
  output : Outport
  wires:
  VCU_MCU1_mux/1 -> output/1
  MCU1HeartBeat/1(output1) -> or1/1
  MCU1HeartBeat/2(output2) -> or2/1
  MCU1HeartBeat/3(output3) -> or3/1
  MCU1HeartBeat/4(output4) -> or4/1
  MCU1HeartBeat/5(output5) -> or5/1
  MCU1HeartBeat/6(output6) -> or6/1
  MCU1HeartBeat/7(output7) -> or7/1
  MCU1HeartBeat/8(output8) -> or8/1
  M2TorqueSet/1(output1) -> or1/2
  M2TorqueSet/2(output2) -> or2/2
  M2TorqueSet/3(output3) -> or3/2
  M2TorqueSet/4(output4) -> or4/2
  M2TorqueSet/5(output5) -> or5/2
  M2TorqueSet/6(output6) -> or6/2
  M2TorqueSet/7(output7) -> or7/2
  M2TorqueSet/8(output8) -> or8/2
  M2SpeedLimit/1(output1) -> or1/3
  M2SpeedLimit/2(output2) -> or2/3
  M2SpeedLimit/3(output3) -> or3/3
  M2SpeedLimit/4(output4) -> or4/3
  M2SpeedLimit/5(output5) -> or5/3
  M2SpeedLimit/6(output6) -> or6/3
  M2SpeedLimit/7(output7) -> or7/3
  M2SpeedLimit/8(output8) -> or8/3
  M2Mode/1(output1) -> or1/4
  M2Mode/2(output2) -> or2/4
  M2Mode/3(output3) -> or3/4
  M2Mode/4(output4) -> or4/4
  M2Mode/5(output5) -> or5/4
  M2Mode/6(output6) -> or6/4
  M2Mode/7(output7) -> or7/4
  M2Mode/8(output8) -> or8/4
  M2Enable/1(output1) -> or1/5
  M2Enable/2(output2) -> or2/5
  M2Enable/3(output3) -> or3/5
  M2Enable/4(output4) -> or4/5
  M2Enable/5(output5) -> or5/5
  M2Enable/6(output6) -> or6/5
  M2Enable/7(output7) -> or7/5
  M2Enable/8(output8) -> or8/5
  M2Drive/1(output1) -> or1/6
  M2Drive/2(output2) -> or2/6
  M2Drive/3(output3) -> or3/6
  M2Drive/4(output4) -> or4/6
  M2Drive/5(output5) -> or5/6
  M2Drive/6(output6) -> or6/6
  M2Drive/7(output7) -> or7/6
  M2Drive/8(output8) -> or8/6
  M1TorqueSet/1(output1) -> or1/7
  M1TorqueSet/2(output2) -> or2/7
  M1TorqueSet/3(output3) -> or3/7
  M1TorqueSet/4(output4) -> or4/7
  M1TorqueSet/5(output5) -> or5/7
  M1TorqueSet/6(output6) -> or6/7
  M1TorqueSet/7(output7) -> or7/7
  M1TorqueSet/8(output8) -> or8/7
  M1SpeedLimit/1(output1) -> or1/8
  M1SpeedLimit/2(output2) -> or2/8
  M1SpeedLimit/3(output3) -> or3/8
  M1SpeedLimit/4(output4) -> or4/8
  M1SpeedLimit/5(output5) -> or5/8
  M1SpeedLimit/6(output6) -> or6/8
  M1SpeedLimit/7(output7) -> or7/8
  M1SpeedLimit/8(output8) -> or8/8
  M1Mode/1(output1) -> or1/9
  M1Mode/2(output2) -> or2/9
  M1Mode/3(output3) -> or3/9
  M1Mode/4(output4) -> or4/9
  M1Mode/5(output5) -> or5/9
  M1Mode/6(output6) -> or6/9
  M1Mode/7(output7) -> or7/9
  M1Mode/8(output8) -> or8/9
  M1Enable/1(output1) -> or1/10
  M1Enable/2(output2) -> or2/10
  M1Enable/3(output3) -> or3/10
  M1Enable/4(output4) -> or4/10
  M1Enable/5(output5) -> or5/10
  M1Enable/6(output6) -> or6/10
  M1Enable/7(output7) -> or7/10
  M1Enable/8(output8) -> or8/10
  M1Drive/1(output1) -> or1/11
  M1Drive/2(output2) -> or2/11
  M1Drive/3(output3) -> or3/11
  M1Drive/4(output4) -> or4/11
  M1Drive/5(output5) -> or5/11
  M1Drive/6(output6) -> or6/11
  M1Drive/7(output7) -> or7/11
  M1Drive/8(output8) -> or8/11
  or1/1 -> Conv1/1
  Conv1/1 -> VCU_MCU1_mux/1
  or2/1 -> Conv2/1
  Conv2/1 -> VCU_MCU1_mux/2
  or3/1 -> Conv3/1
  Conv3/1 -> VCU_MCU1_mux/3
  or4/1 -> Conv4/1
  Conv4/1 -> VCU_MCU1_mux/4
  or5/1 -> Conv5/1
  Conv5/1 -> VCU_MCU1_mux/5
  or6/1 -> Conv6/1
  Conv6/1 -> VCU_MCU1_mux/6
  or7/1 -> Conv7/1
  Conv7/1 -> VCU_MCU1_mux/7
  or8/1 -> Conv8/1
  Conv8/1 -> VCU_MCU1_mux/8
  VCU_MCU1_ID/1 -> VCU_MCU1_ID_Out/1
  VCU_MCU1_DLC/1 -> VCU_MCU1_DLC_Out/1
  MCU1HeartBeat_in/1 -> MCU1HeartBeat/1(MCU1HeartBeat)
  M2TorqueSet_in/1 -> M2TorqueSet/1(M2TorqueSet)
  M2SpeedLimit_in/1 -> M2SpeedLimit/1(M2SpeedLimit)
  M2Mode_in/1 -> M2Mode/1(M2Mode)
  M2Enable_in/1 -> M2Enable/1(M2Enable)
  M2Drive_in/1 -> M2Drive/1(M2Drive)
  M1TorqueSet_in/1 -> M1TorqueSet/1(M1TorqueSet)
  M1SpeedLimit_in/1 -> M1SpeedLimit/1(M1SpeedLimit)
  M1Mode_in/1 -> M1Mode/1(M1Mode)
  M1Enable_in/1 -> M1Enable/1(M1Enable)
  M1Drive_in/1 -> M1Drive/1(M1Drive)

== system DDCU_wxt_v02_forA_LabviewV03/OutputSignalProcess/VCU_MCU1_replace ==
  M2SpeedSet_in : Inport
  M1SpeedSet_in : Inport  Port=2
  MCU1HeartBeat_in : Inport  Port=3
  M2SpeedLimit_in : Inport  Port=4
  M2Mode_in : Inport  Port=5
  M2Enable_in : Inport  Port=6
  M2Drive_in : Inport  Port=7
  M1SpeedLimit_in : Inport  Port=8
  M1Mode_in : Inport  Port=9
  M1Enable_in : Inport  Port=10
  M1Drive_in : Inport  Port=11
  Conv{1..8} (8 alike) : DataTypeConversion
  M1Drive : Subsystem
  M1Enable : Subsystem
  M1Mode : Subsystem
  M1SpeedLimit : Subsystem
  M1SpeedSet : Subsystem
  M2Drive : Subsystem
  M2Enable : Subsystem
  M2Mode : Subsystem
  M2SpeedLimit : Subsystem
  M2SpeedSet : Subsystem
  MCU1HeartBeat : Subsystem
  VCU_MCU1_replace_DLC : Constant  Value=8  OutDataTypeStr=uint8
  VCU_MCU1_replace_DLC_Out : Terminator
  VCU_MCU1_replace_ID : Constant  Value=2348937233  OutDataTypeStr=single
  VCU_MCU1_replace_ID_Out : Terminator
  VCU_MCU1_replace_mux : Mux  Inputs=8
  or{1..8} (8 alike) : simulink/Logic and Bit Operations/Bitwise Operator  logicop=OR  UseBitMask=off  NumInputPorts=11  BitMask=bin2dec('11011001')  BitMaskRealWorld=Stored Integer
  output : Outport
  wires:
  VCU_MCU1_replace_mux/1 -> output/1
  M2SpeedSet/1(output1) -> or1/1
  M2SpeedSet/2(output2) -> or2/1
  M2SpeedSet/3(output3) -> or3/1
  M2SpeedSet/4(output4) -> or4/1
  M2SpeedSet/5(output5) -> or5/1
  M2SpeedSet/6(output6) -> or6/1
  M2SpeedSet/7(output7) -> or7/1
  M2SpeedSet/8(output8) -> or8/1
  M1SpeedSet/1(output1) -> or1/2
  M1SpeedSet/2(output2) -> or2/2
  M1SpeedSet/3(output3) -> or3/2
  M1SpeedSet/4(output4) -> or4/2
  M1SpeedSet/5(output5) -> or5/2
  M1SpeedSet/6(output6) -> or6/2
  M1SpeedSet/7(output7) -> or7/2
  M1SpeedSet/8(output8) -> or8/2
  MCU1HeartBeat/1(output1) -> or1/3
  MCU1HeartBeat/2(output2) -> or2/3
  MCU1HeartBeat/3(output3) -> or3/3
  MCU1HeartBeat/4(output4) -> or4/3
  MCU1HeartBeat/5(output5) -> or5/3
  MCU1HeartBeat/6(output6) -> or6/3
  MCU1HeartBeat/7(output7) -> or7/3
  MCU1HeartBeat/8(output8) -> or8/3
  M2SpeedLimit/1(output1) -> or1/4
  M2SpeedLimit/2(output2) -> or2/4
  M2SpeedLimit/3(output3) -> or3/4
  M2SpeedLimit/4(output4) -> or4/4
  M2SpeedLimit/5(output5) -> or5/4
  M2SpeedLimit/6(output6) -> or6/4
  M2SpeedLimit/7(output7) -> or7/4
  M2SpeedLimit/8(output8) -> or8/4
  M2Mode/1(output1) -> or1/5
  M2Mode/2(output2) -> or2/5
  M2Mode/3(output3) -> or3/5
  M2Mode/4(output4) -> or4/5
  M2Mode/5(output5) -> or5/5
  M2Mode/6(output6) -> or6/5
  M2Mode/7(output7) -> or7/5
  M2Mode/8(output8) -> or8/5
  M2Enable/1(output1) -> or1/6
  M2Enable/2(output2) -> or2/6
  M2Enable/3(output3) -> or3/6
  M2Enable/4(output4) -> or4/6
  M2Enable/5(output5) -> or5/6
  M2Enable/6(output6) -> or6/6
  M2Enable/7(output7) -> or7/6
  M2Enable/8(output8) -> or8/6
  M2Drive/1(output1) -> or1/7
  M2Drive/2(output2) -> or2/7
  M2Drive/3(output3) -> or3/7
  M2Drive/4(output4) -> or4/7
  M2Drive/5(output5) -> or5/7
  M2Drive/6(output6) -> or6/7
  M2Drive/7(output7) -> or7/7
  M2Drive/8(output8) -> or8/7
  M1SpeedLimit/1(output1) -> or1/8
  M1SpeedLimit/2(output2) -> or2/8
  M1SpeedLimit/3(output3) -> or3/8
  M1SpeedLimit/4(output4) -> or4/8
  M1SpeedLimit/5(output5) -> or5/8
  M1SpeedLimit/6(output6) -> or6/8
  M1SpeedLimit/7(output7) -> or7/8
  M1SpeedLimit/8(output8) -> or8/8
  M1Mode/1(output1) -> or1/9
  M1Mode/2(output2) -> or2/9
  M1Mode/3(output3) -> or3/9
  M1Mode/4(output4) -> or4/9
  M1Mode/5(output5) -> or5/9
  M1Mode/6(output6) -> or6/9
  M1Mode/7(output7) -> or7/9
  M1Mode/8(output8) -> or8/9
  M1Enable/1(output1) -> or1/10
  M1Enable/2(output2) -> or2/10
  M1Enable/3(output3) -> or3/10
  M1Enable/4(output4) -> or4/10
  M1Enable/5(output5) -> or5/10
  M1Enable/6(output6) -> or6/10
  M1Enable/7(output7) -> or7/10
  M1Enable/8(output8) -> or8/10
  M1Drive/1(output1) -> or1/11
  M1Drive/2(output2) -> or2/11
  M1Drive/3(output3) -> or3/11
  M1Drive/4(output4) -> or4/11
  M1Drive/5(output5) -> or5/11
  M1Drive/6(output6) -> or6/11
  M1Drive/7(output7) -> or7/11
  M1Drive/8(output8) -> or8/11
  or1/1 -> Conv1/1
  Conv1/1 -> VCU_MCU1_replace_mux/1
  or2/1 -> Conv2/1
  Conv2/1 -> VCU_MCU1_replace_mux/2
  or3/1 -> Conv3/1
  Conv3/1 -> VCU_MCU1_replace_mux/3
  or4/1 -> Conv4/1
  Conv4/1 -> VCU_MCU1_replace_mux/4
  or5/1 -> Conv5/1
  Conv5/1 -> VCU_MCU1_replace_mux/5
  or6/1 -> Conv6/1
  Conv6/1 -> VCU_MCU1_replace_mux/6
  or7/1 -> Conv7/1
  Conv7/1 -> VCU_MCU1_replace_mux/7
  or8/1 -> Conv8/1
  Conv8/1 -> VCU_MCU1_replace_mux/8
  VCU_MCU1_replace_ID/1 -> VCU_MCU1_replace_ID_Out/1
  VCU_MCU1_replace_DLC/1 -> VCU_MCU1_replace_DLC_Out/1
  M2SpeedSet_in/1 -> M2SpeedSet/1(M2SpeedSet)
  M1SpeedSet_in/1 -> M1SpeedSet/1(M1SpeedSet)
  MCU1HeartBeat_in/1 -> MCU1HeartBeat/1(MCU1HeartBeat)
  M2SpeedLimit_in/1 -> M2SpeedLimit/1(M2SpeedLimit)
  M2Mode_in/1 -> M2Mode/1(M2Mode)
  M2Enable_in/1 -> M2Enable/1(M2Enable)
  M2Drive_in/1 -> M2Drive/1(M2Drive)
  M1SpeedLimit_in/1 -> M1SpeedLimit/1(M1SpeedLimit)
  M1Mode_in/1 -> M1Mode/1(M1Mode)
  M1Enable_in/1 -> M1Enable/1(M1Enable)
  M1Drive_in/1 -> M1Drive/1(M1Drive)

== system DDCU_wxt_v02_forA_LabviewV03/OutputSignalProcess/VCU_MCU2 ==
  M3Enable_in : Inport
  M3Mode_in : Inport  Port=2
  M3Drive_in : Inport  Port=3
  M3TorqueSet_in : Inport  Port=4
  M3SpeedLimit_in : Inport  Port=5
  M4Enable_in : Inport  Port=6
  M4Mode_in : Inport  Port=7
  M4Drive_in : Inport  Port=8
  M4TorqueSet_in : Inport  Port=9
  M4SpeedLimit_in : Inport  Port=10
  MCU2HeartBeat_in : Inport  Port=11
  Conv{1..8} (8 alike) : DataTypeConversion
  M3Drive : Subsystem
  M3Enable : Subsystem
  M3Mode : Subsystem
  M3SpeedLimit : Subsystem
  M3TorqueSet : Subsystem
  M4Drive : Subsystem
  M4Enable : Subsystem
  M4Mode : Subsystem
  M4SpeedLimit : Subsystem
  M4TorqueSet : Subsystem
  MCU2HeartBeat : Subsystem
  VCU_MCU2_DLC : Constant  Value=8  OutDataTypeStr=uint8
  VCU_MCU2_DLC_Out : Terminator
  VCU_MCU2_ID : Constant  Value=2348937218  OutDataTypeStr=single
  VCU_MCU2_ID_Out : Terminator
  VCU_MCU2_mux : Mux  Inputs=8
  or{1..8} (8 alike) : simulink/Logic and Bit Operations/Bitwise Operator  logicop=OR  UseBitMask=off  NumInputPorts=11  BitMask=bin2dec('11011001')  BitMaskRealWorld=Stored Integer
  output : Outport
  wires:
  VCU_MCU2_mux/1 -> output/1
  MCU2HeartBeat/1(output1) -> or1/1
  MCU2HeartBeat/2(output2) -> or2/1
  MCU2HeartBeat/3(output3) -> or3/1
  MCU2HeartBeat/4(output4) -> or4/1
  MCU2HeartBeat/5(output5) -> or5/1
  MCU2HeartBeat/6(output6) -> or6/1
  MCU2HeartBeat/7(output7) -> or7/1
  MCU2HeartBeat/8(output8) -> or8/1
  M4TorqueSet/1(output1) -> or1/2
  M4TorqueSet/2(output2) -> or2/2
  M4TorqueSet/3(output3) -> or3/2
  M4TorqueSet/4(output4) -> or4/2
  M4TorqueSet/5(output5) -> or5/2
  M4TorqueSet/6(output6) -> or6/2
  M4TorqueSet/7(output7) -> or7/2
  M4TorqueSet/8(output8) -> or8/2
  M4SpeedLimit/1(output1) -> or1/3
  M4SpeedLimit/2(output2) -> or2/3
  M4SpeedLimit/3(output3) -> or3/3
  M4SpeedLimit/4(output4) -> or4/3
  M4SpeedLimit/5(output5) -> or5/3
  M4SpeedLimit/6(output6) -> or6/3
  M4SpeedLimit/7(output7) -> or7/3
  M4SpeedLimit/8(output8) -> or8/3
  M4Mode/1(output1) -> or1/4
  M4Mode/2(output2) -> or2/4
  M4Mode/3(output3) -> or3/4
  M4Mode/4(output4) -> or4/4
  M4Mode/5(output5) -> or5/4
  M4Mode/6(output6) -> or6/4
  M4Mode/7(output7) -> or7/4
  M4Mode/8(output8) -> or8/4
  M4Enable/1(output1) -> or1/5
  M4Enable/2(output2) -> or2/5
  M4Enable/3(output3) -> or3/5
  M4Enable/4(output4) -> or4/5
  M4Enable/5(output5) -> or5/5
  M4Enable/6(output6) -> or6/5
  M4Enable/7(output7) -> or7/5
  M4Enable/8(output8) -> or8/5
  M4Drive/1(output1) -> or1/6
  M4Drive/2(output2) -> or2/6
  M4Drive/3(output3) -> or3/6
  M4Drive/4(output4) -> or4/6
  M4Drive/5(output5) -> or5/6
  M4Drive/6(output6) -> or6/6
  M4Drive/7(output7) -> or7/6
  M4Drive/8(output8) -> or8/6
  M3TorqueSet/1(output1) -> or1/7
  M3TorqueSet/2(output2) -> or2/7
  M3TorqueSet/3(output3) -> or3/7
  M3TorqueSet/4(output4) -> or4/7
  M3TorqueSet/5(output5) -> or5/7
  M3TorqueSet/6(output6) -> or6/7
  M3TorqueSet/7(output7) -> or7/7
  M3TorqueSet/8(output8) -> or8/7
  M3SpeedLimit/1(output1) -> or1/8
  M3SpeedLimit/2(output2) -> or2/8
  M3SpeedLimit/3(output3) -> or3/8
  M3SpeedLimit/4(output4) -> or4/8
  M3SpeedLimit/5(output5) -> or5/8
  M3SpeedLimit/6(output6) -> or6/8
  M3SpeedLimit/7(output7) -> or7/8
  M3SpeedLimit/8(output8) -> or8/8
  M3Mode/1(output1) -> or1/9
  M3Mode/2(output2) -> or2/9
  M3Mode/3(output3) -> or3/9
  M3Mode/4(output4) -> or4/9
  M3Mode/5(output5) -> or5/9
  M3Mode/6(output6) -> or6/9
  M3Mode/7(output7) -> or7/9
  M3Mode/8(output8) -> or8/9
  M3Enable/1(output1) -> or1/10
  M3Enable/2(output2) -> or2/10
  M3Enable/3(output3) -> or3/10
  M3Enable/4(output4) -> or4/10
  M3Enable/5(output5) -> or5/10
  M3Enable/6(output6) -> or6/10
  M3Enable/7(output7) -> or7/10
  M3Enable/8(output8) -> or8/10
  M3Drive/1(output1) -> or1/11
  M3Drive/2(output2) -> or2/11
  M3Drive/3(output3) -> or3/11
  M3Drive/4(output4) -> or4/11
  M3Drive/5(output5) -> or5/11
  M3Drive/6(output6) -> or6/11
  M3Drive/7(output7) -> or7/11
  M3Drive/8(output8) -> or8/11
  or1/1 -> Conv1/1
  Conv1/1 -> VCU_MCU2_mux/1
  or2/1 -> Conv2/1
  Conv2/1 -> VCU_MCU2_mux/2
  or3/1 -> Conv3/1
  Conv3/1 -> VCU_MCU2_mux/3
  or4/1 -> Conv4/1
  Conv4/1 -> VCU_MCU2_mux/4
  or5/1 -> Conv5/1
  Conv5/1 -> VCU_MCU2_mux/5
  or6/1 -> Conv6/1
  Conv6/1 -> VCU_MCU2_mux/6
  or7/1 -> Conv7/1
  Conv7/1 -> VCU_MCU2_mux/7
  or8/1 -> Conv8/1
  Conv8/1 -> VCU_MCU2_mux/8
  VCU_MCU2_ID/1 -> VCU_MCU2_ID_Out/1
  VCU_MCU2_DLC/1 -> VCU_MCU2_DLC_Out/1
  MCU2HeartBeat_in/1 -> MCU2HeartBeat/1(MCU2HeartBeat)
  M4TorqueSet_in/1 -> M4TorqueSet/1(M4TorqueSet)
  M4SpeedLimit_in/1 -> M4SpeedLimit/1(M4SpeedLimit)
  M4Mode_in/1 -> M4Mode/1(M4Mode)
  M4Enable_in/1 -> M4Enable/1(M4Enable)
  M4Drive_in/1 -> M4Drive/1(M4Drive)
  M3TorqueSet_in/1 -> M3TorqueSet/1(M3TorqueSet)
  M3SpeedLimit_in/1 -> M3SpeedLimit/1(M3SpeedLimit)
  M3Mode_in/1 -> M3Mode/1(M3Mode)
  M3Enable_in/1 -> M3Enable/1(M3Enable)
  M3Drive_in/1 -> M3Drive/1(M3Drive)

== matlab function DDCU_wxt_v02_forA_LabviewV03/MainControl/mode_control/forward/forward/Drive/驱动防滑控制TCS/转向TCS/左转/MATLAB Function1 ==
  data: s_act_lr input; flag_lr output; s_opt_zhuan input; s_opt_zhuan_add input; flag_lr_pre input
function flag_lr = fcn(s_act_lr,s_opt_zhuan,s_opt_zhuan_add,flag_lr_pre)
%#codegen
if s_act_lr>s_opt_zhuan+s_opt_zhuan_add
    flag_lr=1;
elseif s_act_lr<s_opt_zhuan
    flag_lr = 0;
else
    flag_lr=flag_lr_pre;
end
end

== matlab function DDCU_wxt_v02_forA_LabviewV03/MainControl/mode_control/forward/forward/Drive/驱动防滑控制TCS/转向TCS/左转/MATLAB Function3 ==
  data: s_act_rr input; flag_rr output; s_opt_zhuan input; s_opt_zhuan_add input; flag_rr_pre input
function flag_rr = fcn(s_act_rr,s_opt_zhuan,s_opt_zhuan_add,flag_rr_pre)
%#codegen
if s_act_rr>s_opt_zhuan+s_opt_zhuan_add
    flag_rr=1;
elseif s_act_rr<s_opt_zhuan
    flag_rr = 0;
else
    flag_rr=flag_rr_pre;
end
end

== matlab function DDCU_wxt_v02_forA_LabviewV03/MainControl/mode_control/forward/forward/Drive/驱动防滑控制TCS/转向TCS/左转/无滑转/HeartBeat ==
  data: life_pre input; life output
function life = fcn(life_pre)
%#codegen
life=life_pre+1;
if life>15
    life=0;
end
end

== matlab function DDCU_wxt_v02_forA_LabviewV03/MainControl/mode_control/forward/forward/Drive/驱动防滑控制TCS/转向TCS/左转/前轮滑转/HeartBeat ==
  data: life_pre input; life output
function life = fcn(life_pre)
%#codegen
life=life_pre+1;
if life>15
    life=0;
end
end

== matlab function DDCU_wxt_v02_forA_LabviewV03/MainControl/mode_control/forward/forward/Drive/驱动防滑控制TCS/转向TCS/左转/后轮滑转/HeartBeat1 ==
  data: life_pre input; life output
function life = fcn(life_pre)
%#codegen
life=life_pre+1;
if life>15
    life=0;
end
end

== matlab function DDCU_wxt_v02_forA_LabviewV03/MainControl/mode_control/forward/forward/Drive/驱动防滑控制TCS/转向TCS/右转/MATLAB Function ==
  data: s_act_lf input; flag_lf output; s_opt_zhuan input; s_opt_zhuan_add input; flag_lf_pre input
function flag_lf = fcn(s_act_lf,s_opt_zhuan,s_opt_zhuan_add,flag_lf_pre)
%#codegen
if s_act_lf>s_opt_zhuan+s_opt_zhuan_add
    flag_lf=1;
elseif s_act_lf<s_opt_zhuan
    flag_lf = 0;
else
    flag_lf=flag_lf_pre;
end
end

== matlab function DDCU_wxt_v02_forA_LabviewV03/MainControl/mode_control/forward/forward/Drive/驱动防滑控制TCS/转向TCS/右转/MATLAB Function3 ==
  data: s_act_rr input; flag_rr output; s_opt_zhuan input; s_opt_zhuan_add input; flag_rr_pre input
function flag_rr = fcn(s_act_rr,s_opt_zhuan,s_opt_zhuan_add,flag_rr_pre)
%#codegen
if s_act_rr>s_opt_zhuan+s_opt_zhuan_add
    flag_rr=1;
elseif s_act_rr<s_opt_zhuan
    flag_rr = 0;
else
    flag_rr=flag_rr_pre;
end
end

== matlab function DDCU_wxt_v02_forA_LabviewV03/MainControl/mode_control/forward/forward/Drive/驱动防滑控制TCS/转向TCS/右转/前后轮均滑转/HeartBeat1 ==
  data: life_pre input; life output
function life = fcn(life_pre)
%#codegen
life=life_pre+1;
if life>15
    life=0;
end
end

== matlab function DDCU_wxt_v02_forA_LabviewV03/MainControl/mode_control/neutral/neutral/HeartBeat ==
  data: life_pre input; life output
function life = fcn(life_pre)
%#codegen
life=life_pre+1;
if life>15
    life=0;
end
end
